simulink library "PiCar_library"  (R2018a)
settings: Solver=VariableStepAuto  StartTime=0.0  StopTime=10.0  RelTol=1e-3
undefined symbols (not defined in the file or in its folder): gray
libraries: visiontransforms x2, simulink x1, visiontextngfix x1, visionanalysis x1, visionstatistics x1, embdlinuxlib x1
settings Model: Creator=Malte  LastModifiedBy=raspberry

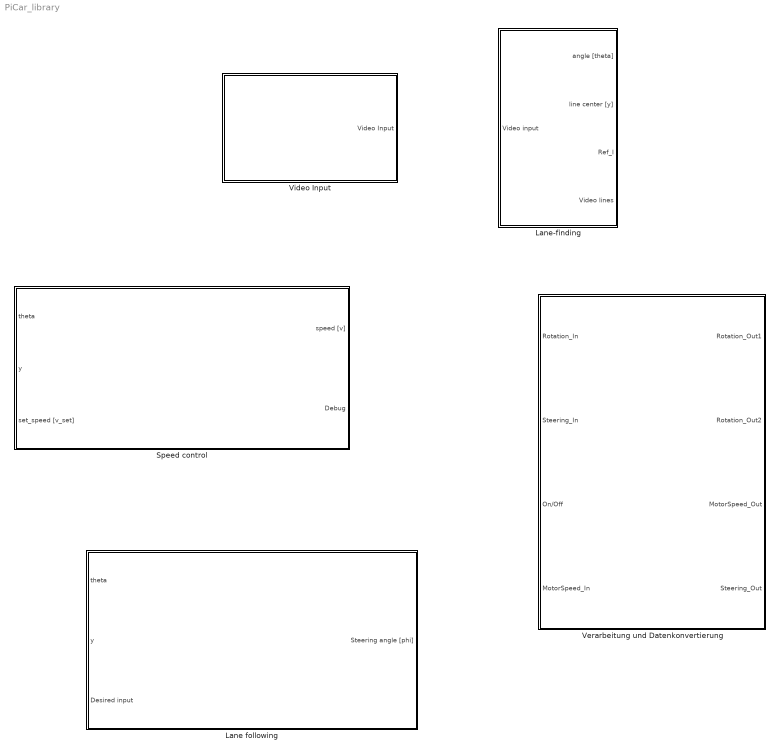
== system PiCar_library ==
  Lane following : Subsystem
  Lane-finding : Subsystem
  Speed control : Subsystem
  Verarbeitung und Datenkonvertierung : Subsystem
  Video Input : Subsystem

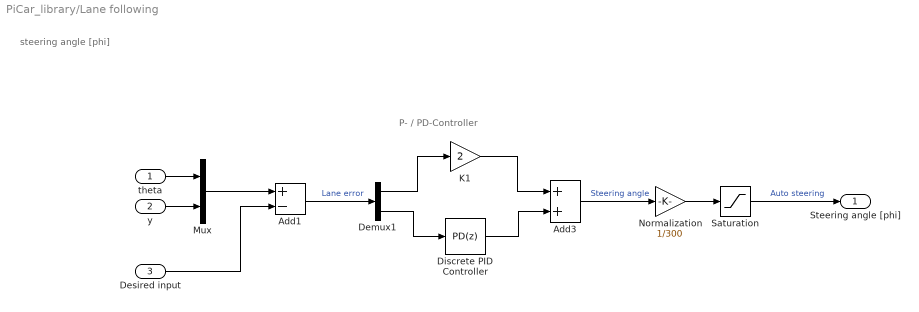
== system PiCar_library/Lane following ==
  note: P- / PD-Controller
  note: steering angle [phi]
  theta : Inport
  y : Inport  Port=2
  Desired input : Inport  Port=3
  Add1 : Sum  Inputs=+-
  Add3 : Sum
  Demux1 : Demux  Outputs=2
  Discrete PID Controller : simulink/Continuous/PID Controller  Controller=PD  TimeDomain=Discrete-time  SampleTime=-1  IntegratorMethod=Forward Euler  FilterMethod=Forward Euler  Form=Parallel  UseFilter=off  ControllerParametersSource=internal  P=18  I=1.5  D=2  N=100  InitialConditionSource=internal  InitialConditionForIntegrator=0  InitialConditionForFilter=0  ExternalReset=none  LimitOutput=off  UpperSaturationLimit=inf  LowerSaturationLimit=-inf  LinearizeAsGain=off  AntiWindupMode=none  Kb=1  TrackingMode=off  Kt=1  PParamMin=[]  PParamMax=[]  IParamMin=[]  IParamMax=[]  DParamMin=[]  DParamMax=[]  NParamMin=[]  NParamMax=[]  KbParamMin=[]  KbParamMax=[]  KtParamMin=[]  KtParamMax=[]  POutMin=[]  POutMax=[]  IOutMin=[]  IOutMax=[]  DOutMin=[]  DOutMax=[]  NOutMin=[]  NOutMax=[]  KbOutMin=[]  KbOutMax=[]  KtOutMin=[]  KtOutMax=[]  IntegratorOutMin=[]  IntegratorOutMax=[]  FilterOutMin=[]  FilterOutMax=[]  SumOutMin=[]  SumOutMax=[]  SumI1OutMin=[]  SumI1OutMax=[]  SumI2OutMin=[]  SumI2OutMax=[]  SumI3OutMin=[]  SumI3OutMax=[]  SumDOutMin=[]  SumDOutMax=[]  SaturationOutMin=[]  SaturationOutMax=[]  IntegratorContinuousStateAttributes=''  IntegratorStateMustResolveToSignalObject=off  IntegratorRTWStateStorageClass=Auto  FilterContinuousStateAttributes=''  FilterStateMustResolveToSignalObject=off  FilterRTWStateStorageClass=Auto  DifferentiatorICPrevScaledInput=0  DifferentiatorOutMin=[]  DifferentiatorOutMax=[]  FilterDiffOutCoefMin=[]  FilterDiffOutCoefMax=[]  SumDenOutMin=[]  SumDenOutMax=[]  SumNumOutMin=[]  SumNumOutMax=[]  ReciprocalOutMin=[]  ReciprocalOutMax=[]  DivideOutMin=[]  DivideOutMax=[]  TunerSelectOption=Transfer Function Based (PID Tuner App)
  K1 : Gain  Gain=2
  Mux : Mux  Inputs=2
  Normalization : Gain  Gain=1/300
  Saturation : Saturate  UpperLimit=1  LowerLimit=-1
  Steering angle [phi] : Outport
  wires:
  K1/1 -> Add3/1
  Demux1/1 -> K1/1
  Add1/1 -> Demux1/1  "Lane error"
  Demux1/2 -> Discrete PID Controller/1
  Discrete PID Controller/1 -> Add3/2
  Add3/1 -> Normalization/1  "Steering angle"
  Saturation/1 -> Steering angle [phi]/1  "Auto steering"
  Normalization/1 -> Saturation/1
  Desired input/1 -> Add1/2
  Mux/1 -> Add1/1
  y/1 -> Mux/2
  theta/1 -> Mux/1

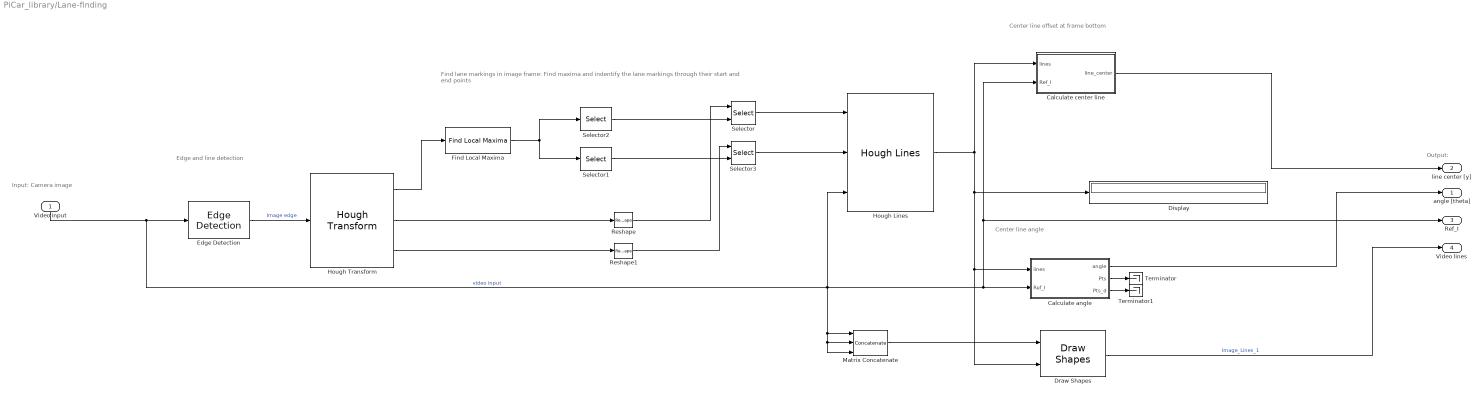
== system PiCar_library/Lane-finding ==
  note: Center line offset at frame bottom
  note: Center line angle
  note: Find lane markings in image frame:
      | Find maxima and indentify the lane markings through their start and end points
  note: Edge and line detection
  note: Input: Camera image
  note: Output:
  Video input : Inport
  Calculate angle : MATLAB Function  TreatAsAtomicUnit=on
  Calculate center line : MATLAB Function  TreatAsAtomicUnit=on
  Display : Display
  Draw Shapes : visiontextngfix/Draw Shapes  shape=Lines  fill=off  lineWidth=1  fillClrSource=Specify via dialog  display=User-specified value  intensity=200  color=[0 0 255]  opacity=0.6  viewport=Entire image  antialiasing=off  inType=Obsolete  imagePorts=One multidimensional signal  prodOutputMode=Binary point scaling  prodOutputWordLength=32  prodOutputFracLength=14  memoryMode=Specify word length  memoryWordLength=16  memoryFracLength=14  roundingMode=Floor  overflowMode=off
      settings: SourceProductName=Computer Vision System Toolbox
  Edge Detection : visionanalysis/Edge Detection  method=Sobel  outputType=Binary image  userDefinedThreshold=off  thresholdSource=Input port  threshold=20  thresholdTuning=4  edgeThinning=off  threshold_canny=[0.25 0.60]  autoPercent=70  sigma=1  roundingMode=Floor  overflowMode=off  prodOutputMode=Binary point scaling  prodOutputWordLength=32  prodOutputFracLength=8  prodOutputSlope=2^-8  accumSlope=2^-8  outputSlope=2^-4
      settings: SourceProductName=Computer Vision System Toolbox  SourceProductBaseCode=VP
  Find Local Maxima : visionstatistics/Find Local Maxima  num_peaks=2  nhood_size=[5 7]  src_thresh=Obsolete9b  src_thresh_inuse=Specify via dialog  threshold=10  inputIsHough=off  dt_peak=uint32  isOutVarDim=on  dt_count=uint32
      settings: SourceProductName=Computer Vision System Toolbox  SourceProductBaseCode=VP
  Hough Lines : visiontransforms/Hough Lines  sineCompMethod=Trigonometric function  thetaRes=pi/180  firstCoeffMode=Specify word length  firstCoeffWordLength=16  firstCoeffFracLength=15  prodOutputMode=Binary point scaling  prodOutputWordLength=32  prodOutputFracLength=16  roundingMode=Nearest  overflowMode=on
      settings: SourceProductName=Computer Vision System Toolbox  SourceProductBaseCode=VP
  Hough Transform : visiontransforms/Hough Transform  theta_res=pi/180  rho_res=1  out_theta_rho=on  outdtmode=double  firstCoeffMode=Binary point scaling  firstCoeffWordLength=16  firstCoeffFracLength=14  secondCoeffMode=Binary point scaling  secondCoeffWordLength=32  secondCoeffFracLength=16  outputMode=Binary point scaling  outputWordLength=16  outputFracLength=0  accumMode=Binary point scaling  accumWordLength=32  accumFracLength=20  prodOutputMode=Binary point scaling  prodOutputWordLength=32  prodOutputFracLength=20  memoryMode=Binary point scaling  memoryWordLength=32  memoryFracLength=16  roundingMode=Nearest  overflowMode=on
      settings: SourceProductName=Computer Vision System Toolbox  SourceProductBaseCode=VP
  Matrix Concatenate : Concatenate  NumInputs=3  Mode=Multidimensional array  ConcatenateDimension=3
  Reshape : Reshape
  Reshape1 : Reshape
  Selector : Selector  IndexOptions=Index vector (port)  Indices=[1 3]  OutputSizes=1
  Selector1 : Selector  NumberOfDimensions=2  InputPortWidth=3  IndexOptions=Select all,Index vector (dialog)  Indices=[1 3],2  OutputSizes=1,1
  Selector2 : Selector  NumberOfDimensions=2  InputPortWidth=3  IndexOptions=Select all,Index vector (dialog)  Indices=[1 3],1  OutputSizes=1,1
  Selector3 : Selector  IndexOptions=Index vector (port)  Indices=[1 3]  OutputSizes=1
  Terminator : Terminator
  Terminator1 : Terminator
  angle [theta] : Outport
  line center [y] : Outport  Port=2
  Ref_I : Outport  Port=3
  Video lines : Outport  Port=4
  wires:
  Calculate angle/2(Pts) -> Terminator/1
  Calculate angle/3(Pts_d) -> Terminator1/1
  Edge Detection/1 -> Hough Transform/1  "Image edge"
  Video input/1 -> Calculate angle/2(Ref_I), Calculate center line/2(Ref_I), Ref_I/1, Hough Lines/3, Matrix Concatenate/1, Matrix Concatenate/2, Matrix Concatenate/3, Edge Detection/1  "video input"
  Hough Transform/2 -> Reshape/1
  Hough Transform/3 -> Reshape1/1
  Hough Transform/1 -> Find Local Maxima/1
  Selector1/1 -> Selector3/2
  Selector2/1 -> Selector/2
  Find Local Maxima/1 -> Selector2/1, Selector1/1
  Selector/1 -> Hough Lines/1
  Reshape/1 -> Selector/1
  Selector3/1 -> Hough Lines/2
  Reshape1/1 -> Selector3/1
  Matrix Concatenate/1 -> Draw Shapes/1
  Calculate angle/1(angle) -> angle [theta]/1
  Draw Shapes/1 -> Video lines/1  "Image_Lines_1"
  Hough Lines/1 -> Calculate center line/1(lines), Display/1, Draw Shapes/2, Calculate angle/1(lines)
  Calculate center line/1(line_center) -> line center [y]/1

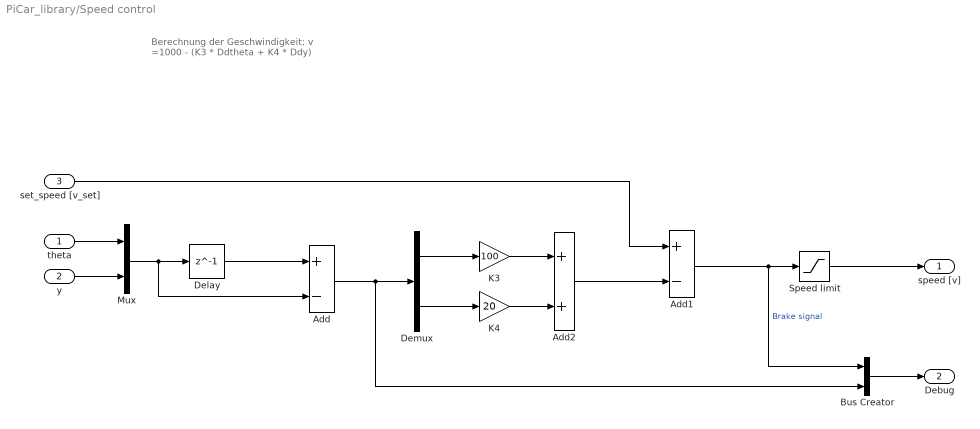
== system PiCar_library/Speed control ==
  note: Berechnung der Geschwindigkeit:
      |
      | v =1000 - (K3 * Ddtheta + K4 * Ddy)
  theta : Inport
  y : Inport  Port=2
  set_speed [v_set] : Inport  Port=3
  Add : Sum  Inputs=+-
  Add1 : Sum  Inputs=+-
  Add2 : Sum
  Bus Creator : BusCreator  Inputs=2
  Delay : Delay  DelayLength=1  InitialCondition=0
  Demux : Demux  Outputs=2
  K3 : Gain  Gain=100
  K4 : Gain  Gain=20
  Mux : Mux  Inputs=2
  Speed limit : Saturate  UpperLimit=0.4  LowerLimit=0
  speed [v] : Outport
  Debug : Outport  Port=2
  wires:
  Mux/1 -> Add/2, Delay/1
  Delay/1 -> Add/1
  Add/1 -> Bus Creator/2, Demux/1
  Demux/1 -> K3/1
  Demux/2 -> K4/1
  Add2/1 -> Add1/2
  Add1/1 -> Bus Creator/1, Speed limit/1  "Brake signal"
  set_speed [v_set]/1 -> Add1/1
  K4/1 -> Add2/2
  K3/1 -> Add2/1
  Bus Creator/1 -> Debug/1
  y/1 -> Mux/2
  theta/1 -> Mux/1
  Speed limit/1 -> speed [v]/1

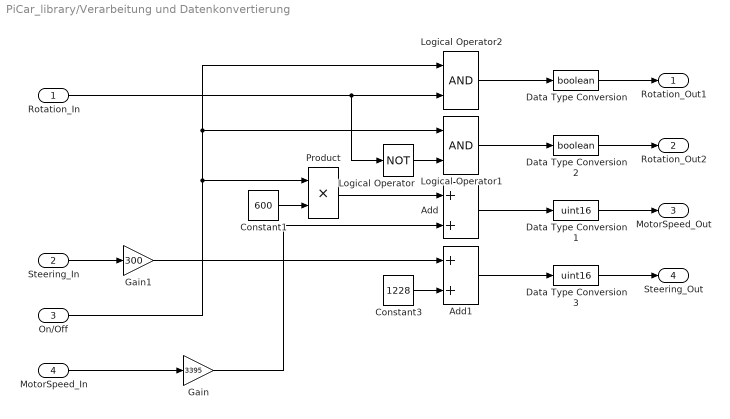
== system PiCar_library/Verarbeitung und Datenkonvertierung ==
  Rotation_In : Inport
  Steering_In : Inport  Port=2
  On/Off : Inport  Port=3
  MotorSpeed_In : Inport  Port=4
  Add : Sum
  Add1 : Sum
  Constant1 : Constant  Value=600
  Constant3 : Constant  Value=1228  OutMin=819  OutMax=1638
  Data Type Conversion : DataTypeConversion  OutDataTypeStr=boolean
  Data Type Conversion1 : DataTypeConversion  OutDataTypeStr=uint16
  Data Type Conversion2 : DataTypeConversion  OutDataTypeStr=boolean
  Data Type Conversion3 : DataTypeConversion  OutDataTypeStr=uint16
  Gain : Gain  Gain=3395
  Gain1 : Gain  Gain=300
  Logical Operator : Logic  Operator=NOT  AllPortsSameDT=off  OutDataTypeStr=boolean
  Logical Operator1 : Logic  AllPortsSameDT=off  OutDataTypeStr=boolean
  Logical Operator2 : Logic  AllPortsSameDT=off  OutDataTypeStr=boolean
  Product : Product
  Rotation_Out1 : Outport
  Rotation_Out2 : Outport  Port=2
  MotorSpeed_Out : Outport  Port=3
  Steering_Out : Outport  Port=4
  wires:
  Logical Operator1/1 -> Data Type Conversion2/1
  Logical Operator2/1 -> Data Type Conversion/1
  Logical Operator/1 -> Logical Operator1/2
  On/Off/1 -> Logical Operator1/1, Logical Operator2/1, Product/1
  Constant3/1 -> Add1/2
  Rotation_In/1 -> Logical Operator/1, Logical Operator2/2
  Add/1 -> Data Type Conversion1/1
  Add1/1 -> Data Type Conversion3/1
  Constant1/1 -> Product/2
  Product/1 -> Add/1
  Data Type Conversion1/1 -> MotorSpeed_Out/1
  Data Type Conversion3/1 -> Steering_Out/1
  Data Type Conversion2/1 -> Rotation_Out2/1
  MotorSpeed_In/1 -> Gain/1
  Data Type Conversion/1 -> Rotation_Out1/1
  Steering_In/1 -> Gain1/1
  Gain/1 -> Add/2
  Gain1/1 -> Add1/1

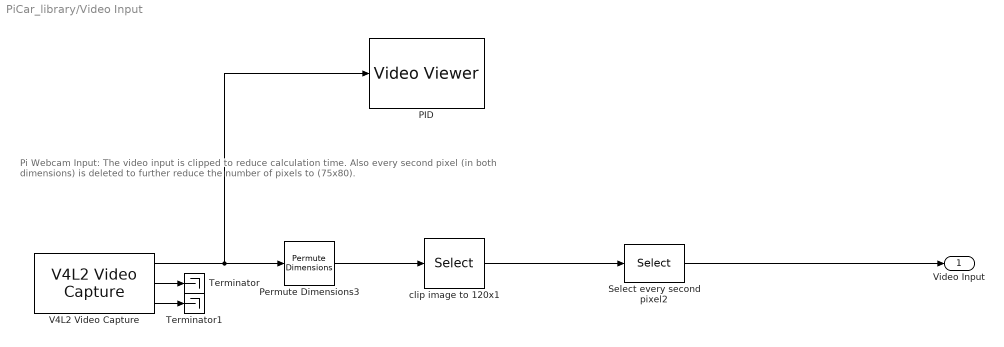
== system PiCar_library/Video Input ==
  note: Pi Webcam Input:
      | The video input is clipped to reduce calculation time. Also every second pixel (in both dimensions) is deleted to further reduce the number of pixels
      | to (75x80).
  PID : VideoViewer  colormapValue=gray(256)  FigPos=[1 1038 1920 938]  OpenAtMdlStart=off
  Permute Dimensions3 : PermuteDimensions
  Select every second pixel2 : Selector  NumberOfDimensions=2  InputPortWidth=3  IndexOptions=Select all,Index vector (dialog)  Indices=[1:2:80],[1:2:160]  OutputSizes=1,1
  Terminator : Terminator
  Terminator1 : Terminator
  V4L2 Video Capture : embdlinuxlib/V4L2 Video Capture  m_devName='/dev/video0'  roi=[0, 0, 640, 480]  imSizeSelection=320x240  imSize=[640, 480]  pixelFormat=YCbCr 4:2:2  pixelOrder=Planar  sampleTime=1/10  simOutput=Colorbars  blockPlatform=Raspberry Pi
      settings: SourceProductName=Simulink Support Package for Raspberry Pi Hardware  SourceProductBaseCode=RASPPI
  clip image to 120x1 : Selector  NumberOfDimensions=2  InputPortWidth=3  IndexOptions=Index vector (dialog),Index vector (dialog)  Indices=[150:1:210],[1:2:320]  OutputSizes=1,1
  Video Input : Outport
  wires:
  V4L2 Video Capture/1 -> Permute Dimensions3/1, PID/1
  Permute Dimensions3/1 -> clip image to 120x1/1
  clip image to 120x1/1 -> Select every second pixel2/1
  V4L2 Video Capture/2 -> Terminator/1
  V4L2 Video Capture/3 -> Terminator1/1
  Select every second pixel2/1 -> Video Input/1

== matlab function PiCar_library/Lane-finding/Calculate angle ==
  data: lines input; angle output; Pts output; Pts_d output; Ref_I input
function [angle, Pts, Pts_d] = angle(lines, Ref_I)

IMAGE_SIZE = size(Ref_I);
IMAGE_HEIGHT = IMAGE_SIZE(1);
IMAGE_WIDTH = IMAGE_SIZE(2);
points = zeros(2,4);

% Sorting the lines
if double(lines(1,1)) < double(lines(2,1))
    points(1,:) = lines(1,:);
    points(2,:) = lines(2,:);
else
    points(1,:) = lines(2,:);
    points(2,:) = lines(1,:);
end

% Calculate the lane center, top and bottom
x_center = double((points(1,:) + points(2,:))/2);

% Calculate the angle of the centerline: 0 -> vertical
angle = atan((x_center(3) - x_center(1))/IMAGE_HEIGHT);

% Auxilliary lines
Pts = int32([x_center(1), 1, x_center(3), 75]);
Pts_d = int32([IMAGE_WIDTH/2, 1, IMAGE_WIDTH/2, 75]);

% angles = atan2d(double((lines(:,1) - lines(:,3))), -double(lines(:,2) - lines(:,4)));

== matlab function PiCar_library/Lane-finding/Calculate center line ==
  data: lines input; line_center output; Ref_I input
function line_center = center(lines, Ref_I)

IMAGE_SIZE = size(Ref_I);
IMAGE_HEIGHT = IMAGE_SIZE(1);
IMAGE_WIDTH = IMAGE_SIZE(2);
points = zeros(2,4);

% Sorting the lines
if double(lines(1,1)) < double(lines(2,1))
    points(1,:) = lines(1,:);
    points(2,:) = lines(2,:);
else
    points(1,:) = lines(2,:);
    points(2,:) = lines(1,:);
end

% Calculate the lane center, top and bottom
x_center = double((points(1,:) + points(2,:))/2);

% Output the lane center at the bottom of the picture
line_center = x_center(3);
